simulink model "simu_circuito"  (R2020b)
settings: Solver=VariableStepAuto  StartTime=0.0  StopTime=0.3  RelTol=1e-3
values from neighbouring files (symbols this model uses):
  C = 10e-6    (= 1e-05)    [par_cir.m]
  L = 1e-3    (= 0.001)    [par_cir.m]
  R1 = 10e3    (= 10000)    [par_cir.m]
  R2 = 1e3    (= 1000)    [par_cir.m]
  R3 = 2.2e3    (= 2200)    [par_cir.m]
settings Model: Creator=Acer  LastModifiedBy=Acer

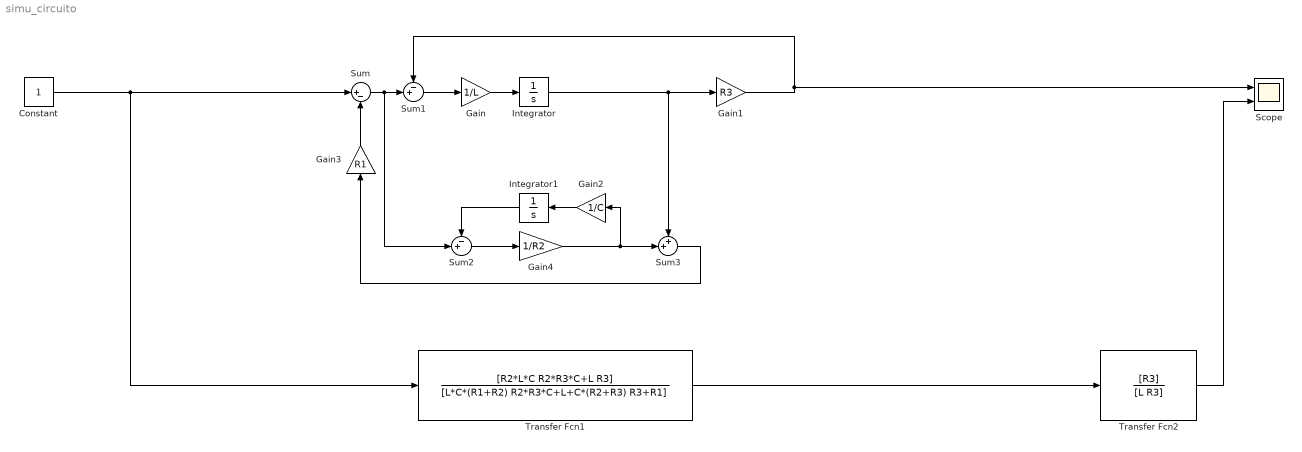
== system simu_circuito ==
  Constant : Constant
  Gain : Gain  Gain=1/L
  Gain1 : Gain  Gain=R3
  Gain2 : Gain  Gain=1/C
  Gain3 : Gain  Gain=R1
  Gain4 : Gain  Gain=1/R2
  Integrator : Integrator
  Integrator1 : Integrator
  Scope : Scope  NumInputPorts=2
  Sum : Sum  Inputs=|+-
  Sum1 : Sum  Inputs=-+|
  Sum2 : Sum  Inputs=-+|
  Sum3 : Sum  Inputs=++|
  Transfer Fcn1 : TransferFcn  Numerator=[R2*L*C R2*R3*C+L R3]  Denominator=[L*C*(R1+R2) R2*R3*C+L+C*(R2+R3) R3+R1]
  Transfer Fcn2 : TransferFcn  Numerator=[R3]  Denominator=[L R3]
  wires:
  Sum/1 -> Sum2/2, Sum1/2
  Gain1/1 -> Scope/1, Sum1/1
  Sum1/1 -> Gain/1
  Gain/1 -> Integrator/1
  Integrator/1 -> Sum3/1, Gain1/1
  Gain2/1 -> Integrator1/1
  Gain3/1 -> Sum/2
  Integrator1/1 -> Sum2/1
  Sum2/1 -> Gain4/1
  Gain4/1 -> Sum3/2, Gain2/1
  Sum3/1 -> Gain3/1
  Transfer Fcn2/1 -> Scope/2
  Constant/1 -> Transfer Fcn1/1, Sum/1
  Transfer Fcn1/1 -> Transfer Fcn2/1
